simulink model "WP2EquipollenzaPolinomi"  (R2023b)
settings: Solver=VariableStepAuto  StartTime=0.0  StopTime=10.0  RelTol=1e-3
undefined symbols (not defined in the file or in its folder): K, x_e
settings Model: Creator=beniaminosquitieri  LastModifiedBy=beniaminosquitieri

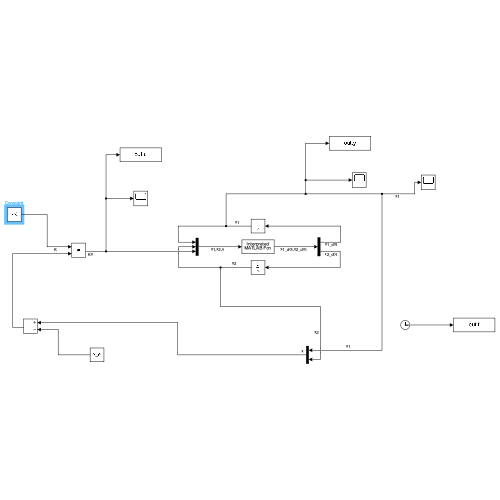
[thumbnail: Simulink's stored preview of the top-level diagram]
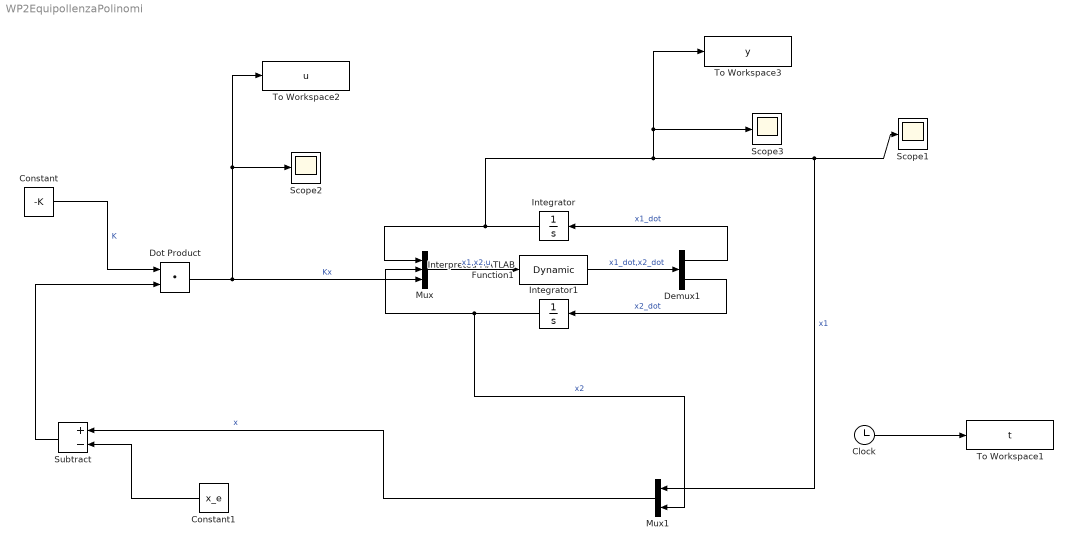
== system WP2EquipollenzaPolinomi ==
  Clock : Clock
  Constant : Constant  Value=-K
  Constant1 : Constant  Value=x_e
  Demux1 : Demux  Outputs=2
  Dot Product : DotProduct  OutDataTypeStr=Inherit: Inherit via internal rule
  Integrator : Integrator
  Integrator1 : Integrator
  Interpreted MATLAB Function1 : MATLABFcn  MATLABFcn=Dynamic  OutputDimensions=2
  Mux : Mux  Inputs=3
  Mux1 : Mux  Inputs=2
  Scope1 : Scope
  Scope2 : Scope
  Scope3 : Scope
  Subtract : Sum  Inputs=+-
  To Workspace1 : ToWorkspace  VariableName=t  SampleTime=-1
  To Workspace2 : ToWorkspace  VariableName=u  SampleTime=-1
  To Workspace3 : ToWorkspace  VariableName=y  SampleTime=-1
  wires:
  Interpreted MATLAB Function1/1 -> Demux1/1  "x1_dot,x2_dot"
  Integrator/1 -> Scope3/1, To Workspace3/1, Mux1/1, Scope1/1, Mux/1  "x1"
  Clock/1 -> To Workspace1/1
  Demux1/1 -> Integrator/1  "x1_dot"
  Constant1/1 -> Subtract/2
  Subtract/1 -> Dot Product/2
  Mux1/1 -> Subtract/1  "x"
  Constant/1 -> Dot Product/1  "K"
  Demux1/2 -> Integrator1/1  "x2_dot"
  Dot Product/1 -> To Workspace2/1, Scope2/1, Mux/3  "Kx"
  Integrator1/1 -> Mux1/2, Mux/2  "x2"
  Mux/1 -> Interpreted MATLAB Function1/1  "x1,x2,u"
